simulink model "dihedral"  (R2024b)
settings: Solver=VariableStepAuto  StartTime=0.0  StopTime=10.0  RelTol=1e-3
undefined symbols (not defined in the file or in its folder): para
settings Model: Creator=feder  LastModifiedBy=feder

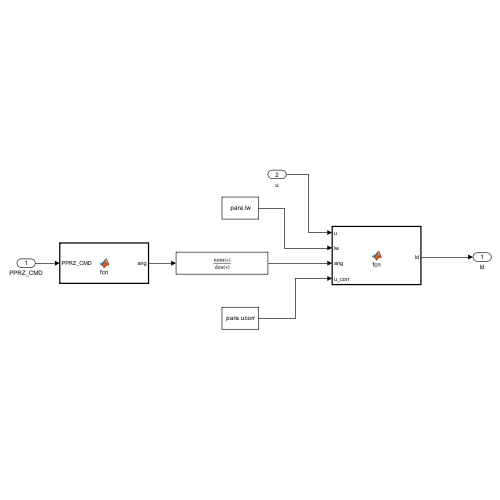
[thumbnail: Simulink's stored preview of the top-level diagram]
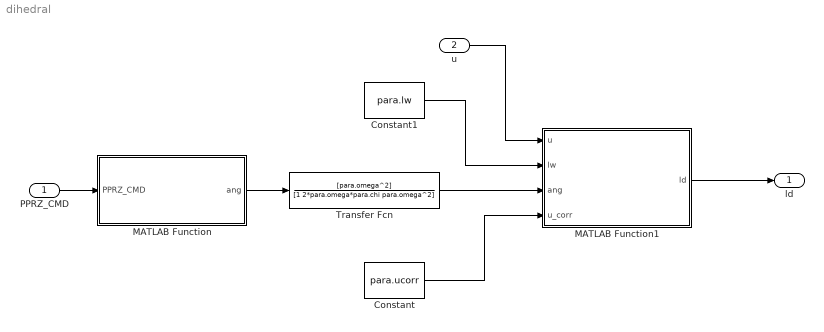
== system dihedral ==
  PPRZ_CMD : Inport
  u : Inport  Port=2
  Constant : Constant  Value=para.ucorr
  Constant1 : Constant  Value=para.lw
  MATLAB Function : MATLAB Function  TreatAsAtomicUnit=on
  MATLAB Function1 : MATLAB Function  TreatAsAtomicUnit=on
  Transfer Fcn : TransferFcn  Numerator=[para.omega^2]  Denominator=[1 2*para.omega*para.chi para.omega^2]
  ld : Outport
  wires:
  PPRZ_CMD/1 -> MATLAB Function/1(PPRZ_CMD)
  MATLAB Function/1(ang) -> Transfer Fcn/1
  Constant/1 -> MATLAB Function1/4(u_corr)
  Transfer Fcn/1 -> MATLAB Function1/3(ang)
  Constant1/1 -> MATLAB Function1/2(lw)
  u/1 -> MATLAB Function1/1(u)
  MATLAB Function1/1(ld) -> ld/1

== matlab function dihedral/MATLAB Function1 ==
  data: u input; lw input; ang input; ld output; u_corr input
function ld = fcn(u, lw, ang, u_corr)


% ang is still in radians
true_ang = (ang + u_corr*u)/180*pi;

ld = lw*sin(true_ang);

== matlab function dihedral/MATLAB Function ==
  data: PPRZ_CMD input; ang output
function ang = fcn(PPRZ_CMD)

ang = - (PPRZ_CMD / 9600*18);
